simulink model "Integration_differentiation"  (R2022b)
settings: Solver=VariableStepAuto  StartTime=0.0  StopTime=100  RelTol=1e-3
libraries: simulink x1
settings Model: Creator=Ayush Pharande  LastModifiedBy=Ayush Pharande

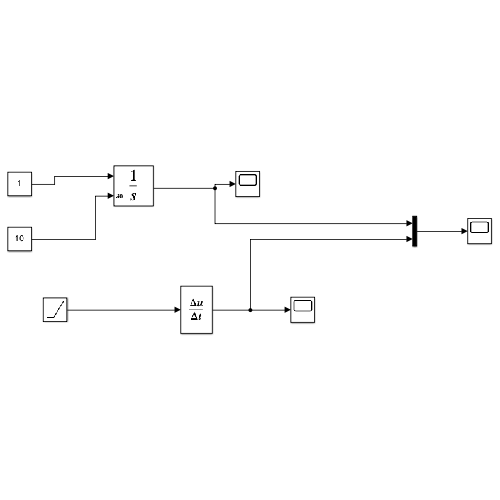
[thumbnail: Simulink's stored preview of the top-level diagram]
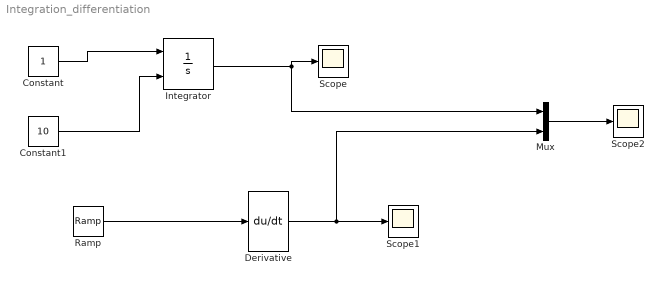
== system Integration_differentiation ==
  Constant : Constant
  Constant1 : Constant  Value=10
  Derivative : Derivative
  Integrator : Integrator  InitialConditionSource=external
  Mux : Mux  Inputs=2
  Ramp : simulink/Sources/Ramp  slope=1  start=0  InitialOutput=0
  Scope : Scope
  Scope1 : Scope
  Scope2 : Scope
  wires:
  Constant/1 -> Integrator/1
  Integrator/1 -> Scope/1, Mux/1
  Derivative/1 -> Mux/2, Scope1/1
  Ramp/1 -> Derivative/1
  Mux/1 -> Scope2/1
  Constant1/1 -> Integrator/2
